simulink model "electromagnet_f"  (R2024a)
settings: Solver=VariableStepAuto  StartTime=0.0  StopTime=te  MaxStep=te/100  RelTol=1e-3
values from neighbouring files (symbols this model uses):
  m = 3    [sim21_solution.m]
  R = 10    [sim21_solution.m]
  U = 230*sqrt(2)    [sim21_solution.m]
  x0 = [0 0]    [sim21_solution.m]
undefined symbols (not defined in the file or in its folder): A, g, lfe, mu0, mur, N, xmin
settings Model: Creator=ocean  LastModifiedBy=ocean

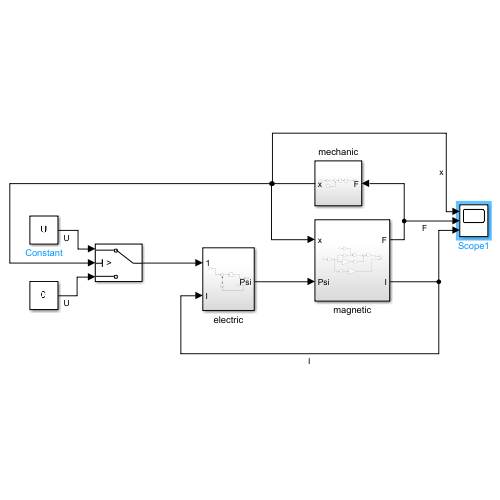
[thumbnail: Simulink's stored preview of the top-level diagram]
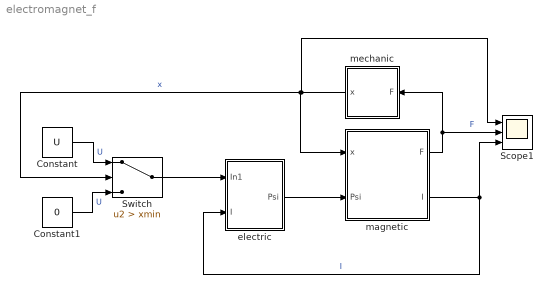
== system electromagnet_f ==
  Constant : Constant  Value=U
  Constant1 : Constant  Value=0
  Scope1 : Scope  NumInputPorts=3
  Switch : Switch  Criteria=u2 > Threshold  Threshold=xmin  SaturateOnIntegerOverflow=off  InputSameDT=off
  electric : Subsystem
  magnetic : Subsystem
  mechanic : Subsystem
  wires:
  magnetic/2(I) -> Scope1/3, electric/2(I)  "I"
  electric/1(Psi) -> magnetic/2(Psi)
  mechanic/1(x) -> Switch/2, magnetic/1(x), Scope1/1  "x"
  magnetic/1(F) -> Scope1/2, mechanic/1(F)  "F"
  Constant/1 -> Switch/1  "U"
  Constant1/1 -> Switch/3  "U"
  Switch/1 -> electric/1(In1)

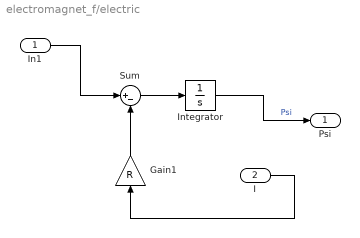
== system electromagnet_f/electric ==
  In1 : Inport
  I : Inport  Port=2
  Gain1 : Gain  Gain=R
  Integrator : Integrator
  Sum : Sum  Inputs=|+-
  Psi : Outport
  wires:
  Gain1/1 -> Sum/2
  Sum/1 -> Integrator/1
  I/1 -> Gain1/1
  In1/1 -> Sum/1
  Integrator/1 -> Psi/1  "Psi"

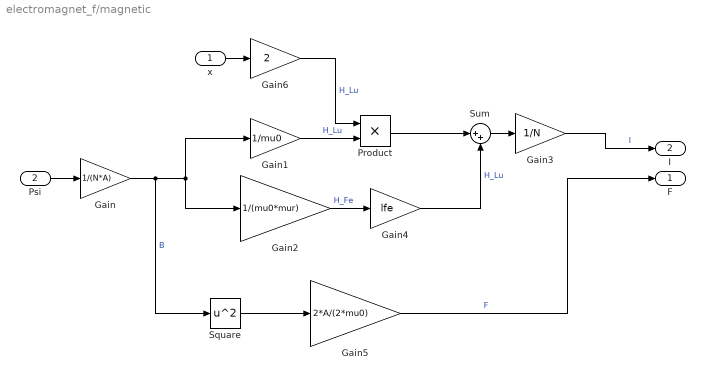
== system electromagnet_f/magnetic ==
  x : Inport
  Psi : Inport  Port=2
  Gain : Gain  Gain=1/(N*A)
  Gain1 : Gain  Gain=1/mu0
  Gain2 : Gain  Gain=1/(mu0*mur)
  Gain3 : Gain  Gain=1/N
  Gain4 : Gain  Gain=lfe
  Gain5 : Gain  Gain=2*A/(2*mu0)
  Gain6 : Gain  Gain=2
  Product : Product
  Square : Math  Operator=square
  Sum : Sum  Inputs=|++
  F : Outport
  I : Outport  Port=2
  wires:
  Product/1 -> Sum/1
  Square/1 -> Gain5/1
  Gain/1 -> Square/1, Gain1/1, Gain2/1  "B"
  Gain4/1 -> Sum/2  "H_Lu"
  Gain2/1 -> Gain4/1  "H_Fe"
  Gain1/1 -> Product/2  "H_Lu"
  Sum/1 -> Gain3/1
  Gain3/1 -> I/1  "I"
  x/1 -> Gain6/1
  Gain5/1 -> F/1  "F"
  Psi/1 -> Gain/1
  Gain6/1 -> Product/1  "H_Lu"

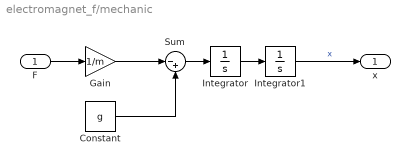
== system electromagnet_f/mechanic ==
  F : Inport
  Constant : Constant  Value=g
  Gain : Gain  Gain=1/m
  Integrator : Integrator
  Integrator1 : Integrator  InitialCondition=x0  LimitOutput=on  LowerSaturationLimit=0
  Sum : Sum  Inputs=|-+
  x : Outport
  wires:
  F/1 -> Gain/1
  Constant/1 -> Sum/2
  Gain/1 -> Sum/1
  Integrator/1 -> Integrator1/1
  Integrator1/1 -> x/1  "x"
  Sum/1 -> Integrator/1
